simulink model "D2C_boucle_vitesse_modelisation"  (R2018a)
settings: Solver=ode45  StartTime=0.0  StopTime=6  FixedStep=0.003  RelTol=1e-3  EnableMultiTasking=on
libraries: simulink x1
settings Model: Creator=Propriétaire  LastModifiedBy=emiliendurif
settings DataIOCC: LimitDataPoints=on  SaveFormat=Array  SignalLoggingSaveFormat=ModelDataLogs
settings OptimizationCC: ExpressionDepthLimit=2147483647  LifeSpan=inf
settings DebuggingCC: UnderspecifiedInitializationDetection=Classic  MergeDetectMultiDrivingBlocksExec=none  SolverPrmCheckMsg=warning  FcnCallInpInsideContextMsg=warning  StateNameClashWarn=warning  SFUnexpectedBacktrackingDiag=warning  SFNoUnconditionalDefaultTransitionDiag=warning  SFExecutionAtInitializationDiag=none
settings HardwareCC: ProdBitPerPointer=32  ProdBitPerSizeT=32  ProdBitPerPtrDiffT=32  ProdLargestAtomicFloat=None  ProdIntDivRoundTo=Undefined  ProdEndianess=Unspecified  ProdWordSize=32  ProdHWDeviceType=32-bit Generic
settings ModelReferenceCC: PropagateSignalLabelsOutOfModel=off
settings CodeAppCC: StateflowObjectComments=on
settings GRTTargetCC: TargetLangStandard=C89/C90 (ANSI)  GeneratePreprocessorConditionals=Disable all  CombineOutputUpdateFcns=off  GRTInterface=on
settings ConfigComp: CovMetricSettings=dw  CovHtmlReporting=on  CovSaveCumulativeToWorkspaceVar=on  CovSaveSingleToWorkspaceVar=on  CovExternalEMLEnable=off

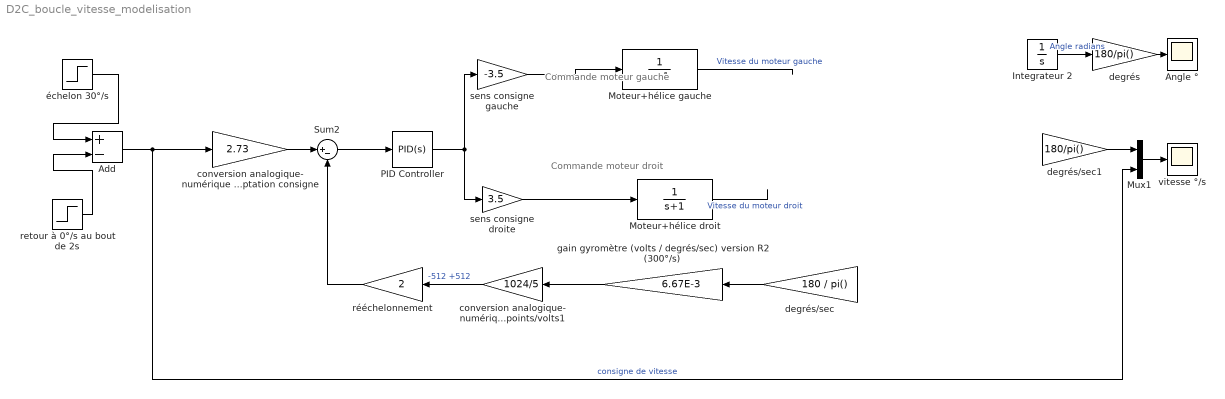
== system D2C_boucle_vitesse_modelisation ==
  note: Commande
      | moteur gauche
  note: Commande
      | moteur droit
  Add : Sum  Inputs=+-
  Angle ° : Scope
  Integrateur 2 : Integrator
  Moteur+hélice droit : TransferFcn  Denominator=[1 1]
  Moteur+hélice gauche : TransferFcn  Denominator=[1 1]
  Mux1 : Mux  Inputs=2
  PID Controller : simulink/Continuous/PID Controller  Controller=PID  TimeDomain=Continuous-time  SampleTime=-1  IntegratorMethod=Forward Euler  FilterMethod=Forward Euler  Form=Parallel  UseFilter=on  ControllerParametersSource=internal  P=1  I=1  D=0  N=100  InitialConditionSource=internal  InitialConditionForIntegrator=0  InitialConditionForFilter=0  ExternalReset=none  LimitOutput=off  UpperSaturationLimit=inf  LowerSaturationLimit=-inf  LinearizeAsGain=on  AntiWindupMode=none  Kb=1  TrackingMode=off  Kt=1  PParamMin=[]  PParamMax=[]  IParamMin=[]  IParamMax=[]  DParamMin=[]  DParamMax=[]  NParamMin=[]  NParamMax=[]  KbParamMin=[]  KbParamMax=[]  KtParamMin=[]  KtParamMax=[]  POutMin=[]  POutMax=[]  IOutMin=[]  IOutMax=[]  DOutMin=[]  DOutMax=[]  NOutMin=[]  NOutMax=[]  KbOutMin=[]  KbOutMax=[]  KtOutMin=[]  KtOutMax=[]  IntegratorOutMin=[]  IntegratorOutMax=[]  FilterOutMin=[]  FilterOutMax=[]  SumOutMin=[]  SumOutMax=[]  SumI1OutMin=[]  SumI1OutMax=[]  SumI2OutMin=[]  SumI2OutMax=[]  SumI3OutMin=[]  SumI3OutMax=[]  SumDOutMin=[]  SumDOutMax=[]  SaturationOutMin=[]  SaturationOutMax=[]  IntegratorContinuousStateAttributes=''  IntegratorStateMustResolveToSignalObject=off  IntegratorRTWStateStorageClass=Auto  FilterContinuousStateAttributes=''  FilterStateMustResolveToSignalObject=off  FilterRTWStateStorageClass=Auto  DifferentiatorICPrevScaledInput=0  DifferentiatorOutMin=[]  DifferentiatorOutMax=[]  FilterDiffOutCoefMin=[]  FilterDiffOutCoefMax=[]  SumDenOutMin=[]  SumDenOutMax=[]  SumNumOutMin=[]  SumNumOutMax=[]  ReciprocalOutMin=[]  ReciprocalOutMax=[]  DivideOutMin=[]  DivideOutMax=[]  TunerSelectOption=Transfer Function Based (PID Tuner App)
  Sum2 : Sum  Inputs=|+-
  conversion analogique- numérique points/volts 15 bits et adaptation consigne : Gain  Gain=2.73
  conversion analogique- numérique points/volts1 : Gain  Gain=1024/5
  degrés : Gain  Gain=180/pi()
  degrés/sec : Gain  Gain=180 / pi()
  degrés/sec1 : Gain  Gain=180/pi()
  gain gyromètre (volts / degrés/sec) version R2 (300°/s) : Gain  Gain=6.67E-3
  retour à 0°/s au bout de 2s : Step  Time=2  After=30  SampleTime=0
  rééchelonnement : Gain  Gain=2
  sens consigne droite : Gain  Gain=3.5
  sens consigne gauche : Gain  Gain=-3.5
  vitesse °/s : Scope
  échelon 30°/s : Step  Time=0  After=30  SampleTime=0
  wires:
  Moteur+hélice gauche/1 -> ?  "Vitesse du moteur gauche"
  Moteur+hélice droit/1 -> ?  "Vitesse du moteur droit"
  gain gyromètre (volts / degrés/sec) version R2 (300°/s)/1 -> conversion analogique- numérique points/volts1/1
  Integrateur 2/1 -> degrés/1  "Angle radians"
  ? -> Integrateur 2/1, degrés/sec1/1, degrés/sec/1  "vitesse angulaire (rad / s)"
  degrés/sec/1 -> gain gyromètre (volts / degrés/sec) version R2 (300°/s)/1
  degrés/1 -> Angle °/1
  Add/1 -> Mux1/2, conversion analogique- numérique points/volts 15 bits et adaptation consigne/1  "consigne de vitesse"
  degrés/sec1/1 -> Mux1/1
  conversion analogique- numérique points/volts1/1 -> rééchelonnement/1  "-512 +512"
  Mux1/1 -> vitesse °/s/1
  sens consigne droite/1 -> Moteur+hélice droit/1
  sens consigne gauche/1 -> Moteur+hélice gauche/1
  échelon 30°/s/1 -> Add/1
  retour à 0°/s au bout de 2s/1 -> Add/2
  rééchelonnement/1 -> Sum2/2
  conversion analogique- numérique points/volts 15 bits et adaptation consigne/1 -> Sum2/1
  Sum2/1 -> PID Controller/1
  PID Controller/1 -> sens consigne gauche/1, sens consigne droite/1
